simulink model "Architecture"  (R2020b)
settings: Solver=VariableStepAuto  StartTime=0.0  StopTime=10.0  RelTol=1e-3
undefined symbols (not defined in the file or in its folder): des, T
libraries: simulink x16
(part 1 of 6)
settings Model: Creator=James Webb  LastModifiedBy=James Webb

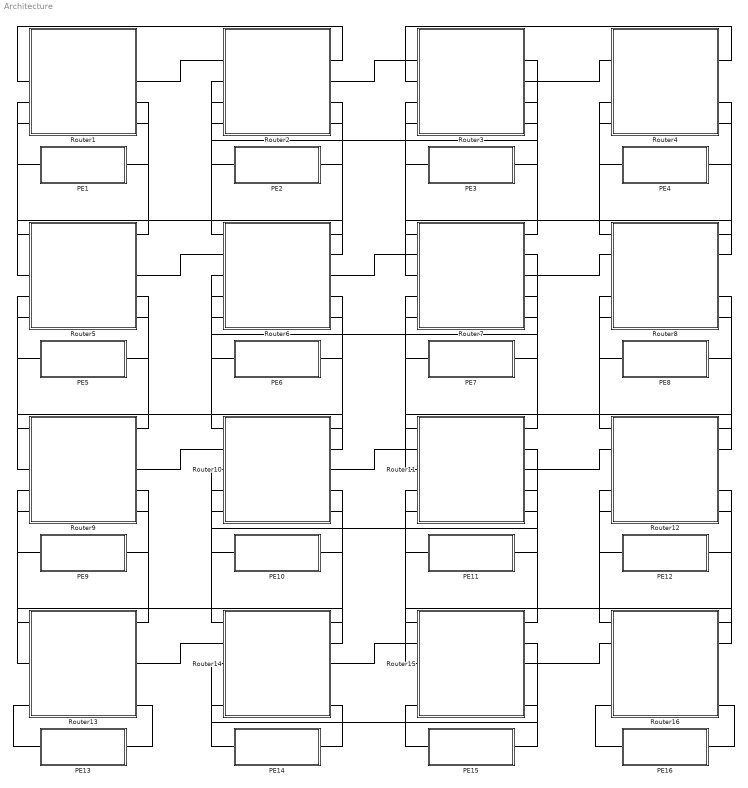
== system Architecture ==
  PE1 : Subsystem  mask{V=[4 16], P=ones(1,2)./2, SELECT=1, ME=1, D=5, SEED=100, tt=Periodic, MINU=10, MAXU=200, REGULAR=T, A=100, B=15, Inst='Inst1', Router='Mean1', Loss='Loss1', N='N1'}
      mask prompts: V "Traffic Pattern"; P "Probabilistic Pattern"; ME "Adress"; D "Startup time"; tt "Traffic Type"; MINU "Min"; MAXU "Max"; REGULAR "T"; A "Lambda 1"; B "Lambda 2"; Inst "Instant delay"; Router "Mean delay"; Loss "Instant number of lost flits"; N "Number of departed flits"
      mask init:
      | set_param([gcb '/Inst'],'VariableName',Inst)
      | set_param([gcb '/Router'],'VariableName',Router)
      | set_param([gcb '/Loss'],'VariableName',Loss)
      | set_param([gcb '/N'],'VariableName',N)
      | %V=[2 7 13];
      | %V=1:20;
      | %V=V(V~=ME);
      mask TypeOptions tt: Periodic | Uniform | MMPP
      mask Callback tt:
      | maskStr = get_param(gcb,'tt');
      | msk = Simulink.Mask.get(gcbh);
      | %p = msk.Parameters;
      | %
      | % P = msk.getParameter('MINU');
      | % U = msk.getParameter('MAXU');
      | % M = msk.getParameter('REGULAR');
      | 
      | P = msk.getDialogControl('Periodic');
      | U = msk.getDialogControl('Uniform');
      | M = msk.getDialogControl('MMPP');
      | 
      | % The pop-up menu is the first mask parameter.
      | %   Check the value selected in the pop-up
      | if strcmp(maskStr(1),'P'),
      | 
      |     % Set the visibility of both parameters on when
      |     %   User-defined is selected in the pop-up.
      |     %set_param(gcb,'MaskValues',{'Default','1','1'})
      |     %set_param(gcb,'MaskVisibilities','off'),
      |     SELECT = 1;
      |     P.Visible= 'on';
      |     U.Visible= 'off';
      |     M.Visible= 'off';
      | 
      | elseif strcmp(maskStr(1),'U'),
      |     P.Visible= 'off';
      |     U.Visible= 'on';
      |     M.Visible= 'off';
      | 
      |     SELECT = 2;
      | else
      |     P.Visible= 'off';
      |     U.Visible= 'off';
      |     M.Visible= 'on';
      | 
      |     SELECT = 3;
      | end
      mask DialogControl DescGroupVar Prompt: Processing Element
      mask DialogControl DescTextVar Prompt: Generates traffic from a given adress using one of three possible traffic patterns: Periodic, Uniform and Markov Modulated Poisson Process.
      mask DialogControl Container8 Prompt: Traffic Routing
      mask DialogControl Container3 Prompt: Parameters
      mask DialogControl Uniform Prompt: Uniform
      mask DialogControl Periodic Prompt: Periodic
      mask DialogControl MMPP Prompt: MMPP
      mask DialogControl Container7 Prompt: Output Variables
  PE10 : Subsystem  mask{V=[3 15], P=ones(1,2)./2, SELECT=1, ME=10, D=5, SEED=100, tt=Periodic, MINU=10, MAXU=200, REGULAR=T, A=100, B=15, Inst='Inst10', Router='Mean10', Loss='Loss10', N='N10'}
      mask prompts: V "Traffic Pattern"; P "Probabilistic Pattern"; ME "Adress"; D "Startup time"; tt "Traffic Type"; MINU "Min"; MAXU "Max"; REGULAR "T"; A "Lambda 1"; B "Lambda 2"; Inst "Instant delay"; Router "Mean delay"; Loss "Instant number of lost flits"; N "Number of departed flits"
      mask init: same as Architecture/PE1
      mask TypeOptions tt: Periodic | Uniform | MMPP
      mask Callback tt:
      | maskStr = get_param(gcb,'tt');
      | msk = Simulink.Mask.get(gcbh);
      | %p = msk.Parameters;
      | %
      | % P = msk.getParameter('MINU');
      | % U = msk.getParameter('MAXU');
      | % M = msk.getParameter('REGULAR');
      | 
      | P = msk.getDialogControl('Periodic');
      | U = msk.getDialogControl('Uniform');
      | M = msk.getDialogControl('MMPP');
      | 
      | % The pop-up menu is the first mask parameter.
      | %   Check the value selected in the pop-up
      | if strcmp(maskStr(1),'P'),
      | 
      |     % Set the visibility of both parameters on when
      |     %   User-defined is selected in the pop-up.
      |     %set_param(gcb,'MaskValues',{'Default','1','1'})
      |     %set_param(gcb,'MaskVisibilities','off'),
      |     SELECT = 1;
      |     P.Visible= 'on';
      |     U.Visible= 'off';
      |     M.Visible= 'off';
      | 
      | elseif strcmp(maskStr(1),'U'),
      |     P.Visible= 'off';
      |     U.Visible= 'on';
      |     M.Visible= 'off';
      | 
      |     SELECT = 2;
      | else
      |     P.Visible= 'off';
      |     U.Visible= 'off';
      |     M.Visible= 'on';
      | 
      |     SELECT = 3;
      | end
      mask DialogControl DescGroupVar Prompt: Processing Element
      mask DialogControl DescTextVar Prompt: Generates traffic from a given adress using one of three possible traffic patterns: Periodic, Uniform and Markov Modulated Poisson Process.
      mask DialogControl Container8 Prompt: Traffic Routing
      mask DialogControl Container3 Prompt: Parameters
      mask DialogControl Uniform Prompt: Uniform
      mask DialogControl Periodic Prompt: Periodic
      mask DialogControl MMPP Prompt: MMPP
      mask DialogControl Container7 Prompt: Output Variables
  PE11 : Subsystem  mask{SELECT=1, ME=11, D=5, SEED=100, tt=Periodic, MINU=10, MAXU=200, REGULAR=T, A=100, B=15, Inst='Inst11', Router='Mean11', Loss='Loss11', N='N11'}
      mask prompts: ME "Adress"; D "Startup time"; tt "Traffic Type"; MINU "Min"; MAXU "Max"; REGULAR "T"; A "Lambda 1"; B "Lambda 2"; Inst "Instant delay"; Router "Mean delay"; Loss "Instant number of lost flits"; N "Number of departed flits"
      mask init: same as Architecture/PE1
      mask TypeOptions tt: Periodic | Uniform | MMPP
      mask Callback tt:
      | maskStr = get_param(gcb,'tt');
      | msk = Simulink.Mask.get(gcbh);
      | %p = msk.Parameters;
      | %
      | % P = msk.getParameter('MINU');
      | % U = msk.getParameter('MAXU');
      | % M = msk.getParameter('REGULAR');
      | 
      | P = msk.getDialogControl('Periodic');
      | U = msk.getDialogControl('Uniform');
      | M = msk.getDialogControl('MMPP');
      | 
      | % The pop-up menu is the first mask parameter.
      | %   Check the value selected in the pop-up
      | if strcmp(maskStr(1),'P'),
      | 
      |     % Set the visibility of both parameters on when
      |     %   User-defined is selected in the pop-up.
      |     %set_param(gcb,'MaskValues',{'Default','1','1'})
      |     %set_param(gcb,'MaskVisibilities','off'),
      |     SELECT = 1;
      |     P.Visible= 'on';
      |     U.Visible= 'off';
      |     M.Visible= 'off';
      | 
      | elseif strcmp(maskStr(1),'U'),
      |     P.Visible= 'off';
      |     U.Visible= 'on';
      |     M.Visible= 'off';
      | 
      |     SELECT = 2;
      | else
      |     P.Visible= 'off';
      |     U.Visible= 'off';
      |     M.Visible= 'on';
      | 
      |     SELECT = 3;
      | end
      mask DialogControl DescGroupVar Prompt: Processing Element
      mask DialogControl DescTextVar Prompt: Generates traffic from a given adress using one of three possible traffic patterns: Periodic, Uniform and Markov Modulated Poisson Process.
      mask DialogControl Container8 Prompt: Traffic Routing
      mask DialogControl Container3 Prompt: Parameters
      mask DialogControl Uniform Prompt: Uniform
      mask DialogControl Periodic Prompt: Periodic
      mask DialogControl MMPP Prompt: MMPP
      mask DialogControl Container7 Prompt: Output Variables
  PE12 : Subsystem  mask{SELECT=1, ME=12, D=5, SEED=100, tt=Periodic, MINU=10, MAXU=200, REGULAR=T, A=100, B=15, Inst='Inst12', Router='Mean12', Loss='Loss12', N='N12'}
      mask prompts: ME "Adress"; D "Startup time"; tt "Traffic Type"; MINU "Min"; MAXU "Max"; REGULAR "T"; A "Lambda 1"; B "Lambda 2"; Inst "Instant delay"; Router "Mean delay"; Loss "Instant number of lost flits"; N "Number of departed flits"
      mask init: same as Architecture/PE1
      mask TypeOptions tt: Periodic | Uniform | MMPP
      mask Callback tt:
      | maskStr = get_param(gcb,'tt');
      | msk = Simulink.Mask.get(gcbh);
      | %p = msk.Parameters;
      | %
      | % P = msk.getParameter('MINU');
      | % U = msk.getParameter('MAXU');
      | % M = msk.getParameter('REGULAR');
      | 
      | P = msk.getDialogControl('Periodic');
      | U = msk.getDialogControl('Uniform');
      | M = msk.getDialogControl('MMPP');
      | 
      | % The pop-up menu is the first mask parameter.
      | %   Check the value selected in the pop-up
      | if strcmp(maskStr(1),'P'),
      | 
      |     % Set the visibility of both parameters on when
      |     %   User-defined is selected in the pop-up.
      |     %set_param(gcb,'MaskValues',{'Default','1','1'})
      |     %set_param(gcb,'MaskVisibilities','off'),
      |     SELECT = 1;
      |     P.Visible= 'on';
      |     U.Visible= 'off';
      |     M.Visible= 'off';
      | 
      | elseif strcmp(maskStr(1),'U'),
      |     P.Visible= 'off';
      |     U.Visible= 'on';
      |     M.Visible= 'off';
      | 
      |     SELECT = 2;
      | else
      |     P.Visible= 'off';
      |     U.Visible= 'off';
      |     M.Visible= 'on';
      | 
      |     SELECT = 3;
      | end
      mask DialogControl DescGroupVar Prompt: Processing Element
      mask DialogControl DescTextVar Prompt: Generates traffic from a given adress using one of three possible traffic patterns: Periodic, Uniform and Markov Modulated Poisson Process.
      mask DialogControl Container8 Prompt: Traffic Routing
      mask DialogControl Container3 Prompt: Parameters
      mask DialogControl Uniform Prompt: Uniform
      mask DialogControl Periodic Prompt: Periodic
      mask DialogControl MMPP Prompt: MMPP
      mask DialogControl Container7 Prompt: Output Variables
  PE13 : Subsystem  mask{SELECT=1, ME=13, D=5, SEED=100, tt=Periodic, MINU=10, MAXU=200, REGULAR=T, A=100, B=15, Inst='Inst13', Router='Mean13', Loss='Loss13', N='N13'}
      mask prompts: ME "Adress"; D "Startup time"; tt "Traffic Type"; MINU "Min"; MAXU "Max"; REGULAR "T"; A "Lambda 1"; B "Lambda 2"; Inst "Instant delay"; Router "Mean delay"; Loss "Instant number of lost flits"; N "Number of departed flits"
      mask init: same as Architecture/PE1
      mask TypeOptions tt: Periodic | Uniform | MMPP
      mask Callback tt:
      | maskStr = get_param(gcb,'tt');
      | msk = Simulink.Mask.get(gcbh);
      | %p = msk.Parameters;
      | %
      | % P = msk.getParameter('MINU');
      | % U = msk.getParameter('MAXU');
      | % M = msk.getParameter('REGULAR');
      | 
      | P = msk.getDialogControl('Periodic');
      | U = msk.getDialogControl('Uniform');
      | M = msk.getDialogControl('MMPP');
      | 
      | % The pop-up menu is the first mask parameter.
      | %   Check the value selected in the pop-up
      | if strcmp(maskStr(1),'P'),
      | 
      |     % Set the visibility of both parameters on when
      |     %   User-defined is selected in the pop-up.
      |     %set_param(gcb,'MaskValues',{'Default','1','1'})
      |     %set_param(gcb,'MaskVisibilities','off'),
      |     SELECT = 1;
      |     P.Visible= 'on';
      |     U.Visible= 'off';
      |     M.Visible= 'off';
      | 
      | elseif strcmp(maskStr(1),'U'),
      |     P.Visible= 'off';
      |     U.Visible= 'on';
      |     M.Visible= 'off';
      | 
      |     SELECT = 2;
      | else
      |     P.Visible= 'off';
      |     U.Visible= 'off';
      |     M.Visible= 'on';
      | 
      |     SELECT = 3;
      | end
      mask DialogControl DescGroupVar Prompt: Processing Element
      mask DialogControl DescTextVar Prompt: Generates traffic from a given adress using one of three possible traffic patterns: Periodic, Uniform and Markov Modulated Poisson Process.
      mask DialogControl Container8 Prompt: Traffic Routing
      mask DialogControl Container3 Prompt: Parameters
      mask DialogControl Uniform Prompt: Uniform
      mask DialogControl Periodic Prompt: Periodic
      mask DialogControl MMPP Prompt: MMPP
      mask DialogControl Container7 Prompt: Output Variables
  PE14 : Subsystem  mask{V=[4 8], P=ones(1,2)./2, SELECT=1, ME=14, D=5, SEED=100, tt=Periodic, MINU=10, MAXU=200, REGULAR=T, A=100, B=15, Inst='Inst14', Router='Mean14', Loss='Loss14', N='N14'}
      mask prompts: V "Traffic Pattern"; P "Probabilistic Pattern"; ME "Adress"; D "Startup time"; tt "Traffic Type"; MINU "Min"; MAXU "Max"; REGULAR "T"; A "Lambda 1"; B "Lambda 2"; Inst "Instant delay"; Router "Mean delay"; Loss "Instant number of lost flits"; N "Number of departed flits"
      mask init: same as Architecture/PE1
      mask TypeOptions tt: Periodic | Uniform | MMPP
      mask Callback tt:
      | maskStr = get_param(gcb,'tt');
      | msk = Simulink.Mask.get(gcbh);
      | %p = msk.Parameters;
      | %
      | % P = msk.getParameter('MINU');
      | % U = msk.getParameter('MAXU');
      | % M = msk.getParameter('REGULAR');
      | 
      | P = msk.getDialogControl('Periodic');
      | U = msk.getDialogControl('Uniform');
      | M = msk.getDialogControl('MMPP');
      | 
      | % The pop-up menu is the first mask parameter.
      | %   Check the value selected in the pop-up
      | if strcmp(maskStr(1),'P'),
      | 
      |     % Set the visibility of both parameters on when
      |     %   User-defined is selected in the pop-up.
      |     %set_param(gcb,'MaskValues',{'Default','1','1'})
      |     %set_param(gcb,'MaskVisibilities','off'),
      |     SELECT = 1;
      |     P.Visible= 'on';
      |     U.Visible= 'off';
      |     M.Visible= 'off';
      | 
      | elseif strcmp(maskStr(1),'U'),
      |     P.Visible= 'off';
      |     U.Visible= 'on';
      |     M.Visible= 'off';
      | 
      |     SELECT = 2;
      | else
      |     P.Visible= 'off';
      |     U.Visible= 'off';
      |     M.Visible= 'on';
      | 
      |     SELECT = 3;
      | end
      mask DialogControl DescGroupVar Prompt: Processing Element
      mask DialogControl DescTextVar Prompt: Generates traffic from a given adress using one of three possible traffic patterns: Periodic, Uniform and Markov Modulated Poisson Process.
      mask DialogControl Container8 Prompt: Traffic Routing
      mask DialogControl Container3 Prompt: Parameters
      mask DialogControl Uniform Prompt: Uniform
      mask DialogControl Periodic Prompt: Periodic
      mask DialogControl MMPP Prompt: MMPP
      mask DialogControl Container7 Prompt: Output Variables
  PE15 : Subsystem  mask{SELECT=1, DST1=[2], ME=15, D=5, SEED=100, tt=Periodic, MINU=10, MAXU=200, REGULAR=T, A=100, B=15, Inst='Inst15', Router='Mean15', Loss='Loss15', N='N15'}
      mask prompts: DST1 "Destino"; ME "Adress"; D "Startup time"; tt "Traffic Type"; MINU "Min"; MAXU "Max"; REGULAR "T"; A "Lambda 1"; B "Lambda 2"; Inst "Instant delay"; Router "Mean delay"; Loss "Instant number of lost flits"; N "Number of departed flits"
      mask init: same as Architecture/PE1
      mask TypeOptions tt: Periodic | Uniform | MMPP
      mask Callback tt:
      | maskStr = get_param(gcb,'tt');
      | msk = Simulink.Mask.get(gcbh);
      | %p = msk.Parameters;
      | %
      | % P = msk.getParameter('MINU');
      | % U = msk.getParameter('MAXU');
      | % M = msk.getParameter('REGULAR');
      | 
      | P = msk.getDialogControl('Periodic');
      | U = msk.getDialogControl('Uniform');
      | M = msk.getDialogControl('MMPP');
      | 
      | % The pop-up menu is the first mask parameter.
      | %   Check the value selected in the pop-up
      | if strcmp(maskStr(1),'P'),
      | 
      |     % Set the visibility of both parameters on when
      |     %   User-defined is selected in the pop-up.
      |     %set_param(gcb,'MaskValues',{'Default','1','1'})
      |     %set_param(gcb,'MaskVisibilities','off'),
      |     SELECT = 1;
      |     P.Visible= 'on';
      |     U.Visible= 'off';
      |     M.Visible= 'off';
      | 
      | elseif strcmp(maskStr(1),'U'),
      |     P.Visible= 'off';
      |     U.Visible= 'on';
      |     M.Visible= 'off';
      | 
      |     SELECT = 2;
      | else
      |     P.Visible= 'off';
      |     U.Visible= 'off';
      |     M.Visible= 'on';
      | 
      |     SELECT = 3;
      | end
      mask DialogControl DescGroupVar Prompt: Processing Element
      mask DialogControl DescTextVar Prompt: Generates traffic from a given adress using one of three possible traffic patterns: Periodic, Uniform and Markov Modulated Poisson Process.
      mask DialogControl Container8 Prompt: Traffic Routing
      mask DialogControl Container3 Prompt: Parameters
      mask DialogControl Uniform Prompt: Uniform
      mask DialogControl Periodic Prompt: Periodic
      mask DialogControl MMPP Prompt: MMPP
      mask DialogControl Container7 Prompt: Output Variables
  PE16 : Subsystem  mask{SELECT=1, DST1=[2], ME=16, D=5, SEED=100, tt=Periodic, MINU=10, MAXU=200, REGULAR=T, A=100, B=15, Inst='Inst16', Router='Mean16', Loss='Loss16', N='N16'}
      mask prompts: DST1 "Destino"; ME "Adress"; D "Startup time"; tt "Traffic Type"; MINU "Min"; MAXU "Max"; REGULAR "T"; A "Lambda 1"; B "Lambda 2"; Inst "Instant delay"; Router "Mean delay"; Loss "Instant number of lost flits"; N "Number of departed flits"
      mask init: same as Architecture/PE1
      mask TypeOptions tt: Periodic | Uniform | MMPP
      mask Callback tt:
      | maskStr = get_param(gcb,'tt');
      | msk = Simulink.Mask.get(gcbh);
      | %p = msk.Parameters;
      | %
      | % P = msk.getParameter('MINU');
      | % U = msk.getParameter('MAXU');
      | % M = msk.getParameter('REGULAR');
      | 
      | P = msk.getDialogControl('Periodic');
      | U = msk.getDialogControl('Uniform');
      | M = msk.getDialogControl('MMPP');
      | 
      | % The pop-up menu is the first mask parameter.
      | %   Check the value selected in the pop-up
      | if strcmp(maskStr(1),'P'),
      | 
      |     % Set the visibility of both parameters on when
      |     %   User-defined is selected in the pop-up.
      |     %set_param(gcb,'MaskValues',{'Default','1','1'})
      |     %set_param(gcb,'MaskVisibilities','off'),
      |     SELECT = 1;
      |     P.Visible= 'on';
      |     U.Visible= 'off';
      |     M.Visible= 'off';
      | 
      | elseif strcmp(maskStr(1),'U'),
      |     P.Visible= 'off';
      |     U.Visible= 'on';
      |     M.Visible= 'off';
      | 
      |     SELECT = 2;
      | else
      |     P.Visible= 'off';
      |     U.Visible= 'off';
      |     M.Visible= 'on';
      | 
      |     SELECT = 3;
      | end
      mask DialogControl DescGroupVar Prompt: Processing Element
      mask DialogControl DescTextVar Prompt: Generates traffic from a given adress using one of three possible traffic patterns: Periodic, Uniform and Markov Modulated Poisson Process.
      mask DialogControl Container8 Prompt: Traffic Routing
      mask DialogControl Container3 Prompt: Parameters
      mask DialogControl Uniform Prompt: Uniform
      mask DialogControl Periodic Prompt: Periodic
      mask DialogControl MMPP Prompt: MMPP
      mask DialogControl Container7 Prompt: Output Variables
  PE2 : Subsystem  mask{V=[3 7 8 9 15], P=ones(1,5)./5, SELECT=1, ME=2, D=5, SEED=100, tt=Periodic, MINU=10, MAXU=200, REGULAR=T, A=100, B=15, Inst='Inst2', Router='Mean2', Loss='Loss2', N='N2'}
      mask prompts: V "Traffic Pattern"; P "Probabilistic Pattern"; ME "Adress"; D "Startup time"; tt "Traffic Type"; MINU "Min"; MAXU "Max"; REGULAR "T"; A "Lambda 1"; B "Lambda 2"; Inst "Instant delay"; Router "Mean delay"; Loss "Instant number of lost flits"; N "Number of departed flits"
      mask init: same as Architecture/PE1
      mask TypeOptions tt: Periodic | Uniform | MMPP
      mask Callback tt:
      | maskStr = get_param(gcb,'tt');
      | msk = Simulink.Mask.get(gcbh);
      | %p = msk.Parameters;
      | %
      | % P = msk.getParameter('MINU');
      | % U = msk.getParameter('MAXU');
      | % M = msk.getParameter('REGULAR');
      | 
      | P = msk.getDialogControl('Periodic');
      | U = msk.getDialogControl('Uniform');
      | M = msk.getDialogControl('MMPP');
      | 
      | % The pop-up menu is the first mask parameter.
      | %   Check the value selected in the pop-up
      | if strcmp(maskStr(1),'P'),
      | 
      |     % Set the visibility of both parameters on when
      |     %   User-defined is selected in the pop-up.
      |     %set_param(gcb,'MaskValues',{'Default','1','1'})
      |     %set_param(gcb,'MaskVisibilities','off'),
      |     SELECT = 1;
      |     P.Visible= 'on';
      |     U.Visible= 'off';
      |     M.Visible= 'off';
      | 
      | elseif strcmp(maskStr(1),'U'),
      |     P.Visible= 'off';
      |     U.Visible= 'on';
      |     M.Visible= 'off';
      | 
      |     SELECT = 2;
      | else
      |     P.Visible= 'off';
      |     U.Visible= 'off';
      |     M.Visible= 'on';
      | 
      |     SELECT = 3;
      | end
      mask DialogControl DescGroupVar Prompt: Processing Element
      mask DialogControl DescTextVar Prompt: Generates traffic from a given adress using one of three possible traffic patterns: Periodic, Uniform and Markov Modulated Poisson Process.
      mask DialogControl Container8 Prompt: Traffic Routing
      mask DialogControl Container3 Prompt: Parameters
      mask DialogControl Uniform Prompt: Uniform
      mask DialogControl Periodic Prompt: Periodic
      mask DialogControl MMPP Prompt: MMPP
      mask DialogControl Container7 Prompt: Output Variables
  PE3 : Subsystem  mask{SELECT=1, DST1=[2], ME=3, D=5, SEED=100, tt=Periodic, MINU=10, MAXU=200, REGULAR=T, A=100, B=15, Inst='Inst3', Router='Mean3', Loss='Loss3', N='N3'}
      mask prompts: DST1 "Destino"; ME "Adress"; D "Startup time"; tt "Traffic Type"; MINU "Min"; MAXU "Max"; REGULAR "T"; A "Lambda 1"; B "Lambda 2"; Inst "Instant delay"; Router "Mean delay"; Loss "Instant number of lost flits"; N "Number of departed flits"
      mask init: same as Architecture/PE1
      mask TypeOptions tt: Periodic | Uniform | MMPP
      mask Callback tt:
      | maskStr = get_param(gcb,'tt');
      | msk = Simulink.Mask.get(gcbh);
      | %p = msk.Parameters;
      | %
      | % P = msk.getParameter('MINU');
      | % U = msk.getParameter('MAXU');
      | % M = msk.getParameter('REGULAR');
      | 
      | P = msk.getDialogControl('Periodic');
      | U = msk.getDialogControl('Uniform');
      | M = msk.getDialogControl('MMPP');
      | 
      | % The pop-up menu is the first mask parameter.
      | %   Check the value selected in the pop-up
      | if strcmp(maskStr(1),'P'),
      | 
      |     % Set the visibility of both parameters on when
      |     %   User-defined is selected in the pop-up.
      |     %set_param(gcb,'MaskValues',{'Default','1','1'})
      |     %set_param(gcb,'MaskVisibilities','off'),
      |     SELECT = 1;
      |     P.Visible= 'on';
      |     U.Visible= 'off';
      |     M.Visible= 'off';
      | 
      | elseif strcmp(maskStr(1),'U'),
      |     P.Visible= 'off';
      |     U.Visible= 'on';
      |     M.Visible= 'off';
      | 
      |     SELECT = 2;
      | else
      |     P.Visible= 'off';
      |     U.Visible= 'off';
      |     M.Visible= 'on';
      | 
      |     SELECT = 3;
      | end
      mask DialogControl DescGroupVar Prompt: Processing Element
      mask DialogControl DescTextVar Prompt: Generates traffic from a given adress using one of three possible traffic patterns: Periodic, Uniform and Markov Modulated Poisson Process.
      mask DialogControl Container8 Prompt: Traffic Routing
      mask DialogControl Container3 Prompt: Parameters
      mask DialogControl Uniform Prompt: Uniform
      mask DialogControl Periodic Prompt: Periodic
      mask DialogControl MMPP Prompt: MMPP
      mask DialogControl Container7 Prompt: Output Variables
  PE4 : Subsystem  mask{SELECT=1, DST1=[7], ME=4, D=5, SEED=100, tt=Periodic, MINU=10, MAXU=200, REGULAR=T, A=100, B=15, Inst='Inst4', Router='Mean4', Loss='Loss4', N='N4'}
      mask prompts: DST1 "Destino"; ME "Adress"; D "Startup time"; tt "Traffic Type"; MINU "Min"; MAXU "Max"; REGULAR "T"; A "Lambda 1"; B "Lambda 2"; Inst "Instant delay"; Router "Mean delay"; Loss "Instant number of lost flits"; N "Number of departed flits"
      mask init: same as Architecture/PE1
      mask TypeOptions tt: Periodic | Uniform | MMPP
      mask Callback tt:
      | maskStr = get_param(gcb,'tt');
      | msk = Simulink.Mask.get(gcbh);
      | %p = msk.Parameters;
      | %
      | % P = msk.getParameter('MINU');
      | % U = msk.getParameter('MAXU');
      | % M = msk.getParameter('REGULAR');
      | 
      | P = msk.getDialogControl('Periodic');
      | U = msk.getDialogControl('Uniform');
      | M = msk.getDialogControl('MMPP');
      | 
      | % The pop-up menu is the first mask parameter.
      | %   Check the value selected in the pop-up
      | if strcmp(maskStr(1),'P'),
      | 
      |     % Set the visibility of both parameters on when
      |     %   User-defined is selected in the pop-up.
      |     %set_param(gcb,'MaskValues',{'Default','1','1'})
      |     %set_param(gcb,'MaskVisibilities','off'),
      |     SELECT = 1;
      |     P.Visible= 'on';
      |     U.Visible= 'off';
      |     M.Visible= 'off';
      | 
      | elseif strcmp(maskStr(1),'U'),
      |     P.Visible= 'off';
      |     U.Visible= 'on';
      |     M.Visible= 'off';
      | 
      |     SELECT = 2;
      | else
      |     P.Visible= 'off';
      |     U.Visible= 'off';
      |     M.Visible= 'on';
      | 
      |     SELECT = 3;
      | end
      mask DialogControl DescGroupVar Prompt: Processing Element
      mask DialogControl DescTextVar Prompt: Generates traffic from a given adress using one of three possible traffic patterns: Periodic, Uniform and Markov Modulated Poisson Process.
      mask DialogControl Container8 Prompt: Traffic Routing
      mask DialogControl Container3 Prompt: Parameters
      mask DialogControl Uniform Prompt: Uniform
      mask DialogControl Periodic Prompt: Periodic
      mask DialogControl MMPP Prompt: MMPP
      mask DialogControl Container7 Prompt: Output Variables
  PE5 : Subsystem  mask{SELECT=1, ME=5, D=5, SEED=100, tt=Periodic, MINU=10, MAXU=200, REGULAR=T, A=100, B=15, Inst='Inst5', Router='Mean5', Loss='Loss5', N='N5'}
      mask prompts: ME "Adress"; D "Startup time"; tt "Traffic Type"; MINU "Min"; MAXU "Max"; REGULAR "T"; A "Lambda 1"; B "Lambda 2"; Inst "Instant delay"; Router "Mean delay"; Loss "Instant number of lost flits"; N "Number of departed flits"
      mask init: same as Architecture/PE1
      mask TypeOptions tt: Periodic | Uniform | MMPP
      mask Callback tt:
      | maskStr = get_param(gcb,'tt');
      | msk = Simulink.Mask.get(gcbh);
      | %p = msk.Parameters;
      | %
      | % P = msk.getParameter('MINU');
      | % U = msk.getParameter('MAXU');
      | % M = msk.getParameter('REGULAR');
      | 
      | P = msk.getDialogControl('Periodic');
      | U = msk.getDialogControl('Uniform');
      | M = msk.getDialogControl('MMPP');
      | 
      | % The pop-up menu is the first mask parameter.
      | %   Check the value selected in the pop-up
      | if strcmp(maskStr(1),'P'),
      | 
      |     % Set the visibility of both parameters on when
      |     %   User-defined is selected in the pop-up.
      |     %set_param(gcb,'MaskValues',{'Default','1','1'})
      |     %set_param(gcb,'MaskVisibilities','off'),
      |     SELECT = 1;
      |     P.Visible= 'on';
      |     U.Visible= 'off';
      |     M.Visible= 'off';
      | 
      | elseif strcmp(maskStr(1),'U'),
      |     P.Visible= 'off';
      |     U.Visible= 'on';
      |     M.Visible= 'off';
      | 
      |     SELECT = 2;
      | else
      |     P.Visible= 'off';
      |     U.Visible= 'off';
      |     M.Visible= 'on';
      | 
      |     SELECT = 3;
      | end
      mask DialogControl DescGroupVar Prompt: Processing Element
      mask DialogControl DescTextVar Prompt: Generates traffic from a given adress using one of three possible traffic patterns: Periodic, Uniform and Markov Modulated Poisson Process.
      mask DialogControl Container8 Prompt: Traffic Routing
      mask DialogControl Container3 Prompt: Parameters
      mask DialogControl Uniform Prompt: Uniform
      mask DialogControl Periodic Prompt: Periodic
      mask DialogControl MMPP Prompt: MMPP
      mask DialogControl Container7 Prompt: Output Variables
  PE6 : Subsystem  mask{SELECT=1, DST1=[3], ME=6, D=5, SEED=100, tt=Periodic, MINU=10, MAXU=200, REGULAR=T, A=100, B=15, Inst='Inst6', Router='Mean6', Loss='Loss6', N='N6'}
      mask prompts: DST1 "Destino"; ME "Adress"; D "Startup time"; tt "Traffic Type"; MINU "Min"; MAXU "Max"; REGULAR "T"; A "Lambda 1"; B "Lambda 2"; Inst "Instant delay"; Router "Mean delay"; Loss "Instant number of lost flits"; N "Number of departed flits"
      mask init: same as Architecture/PE1
      mask TypeOptions tt: Periodic | Uniform | MMPP
      mask Callback tt:
      | maskStr = get_param(gcb,'tt');
      | msk = Simulink.Mask.get(gcbh);
      | %p = msk.Parameters;
      | %
      | % P = msk.getParameter('MINU');
      | % U = msk.getParameter('MAXU');
      | % M = msk.getParameter('REGULAR');
      | 
      | P = msk.getDialogControl('Periodic');
      | U = msk.getDialogControl('Uniform');
      | M = msk.getDialogControl('MMPP');
      | 
      | % The pop-up menu is the first mask parameter.
      | %   Check the value selected in the pop-up
      | if strcmp(maskStr(1),'P'),
      | 
      |     % Set the visibility of both parameters on when
      |     %   User-defined is selected in the pop-up.
      |     %set_param(gcb,'MaskValues',{'Default','1','1'})
      |     %set_param(gcb,'MaskVisibilities','off'),
      |     SELECT = 1;
      |     P.Visible= 'on';
      |     U.Visible= 'off';
      |     M.Visible= 'off';
      | 
      | elseif strcmp(maskStr(1),'U'),
      |     P.Visible= 'off';
      |     U.Visible= 'on';
      |     M.Visible= 'off';
      | 
      |     SELECT = 2;
      | else
      |     P.Visible= 'off';
      |     U.Visible= 'off';
      |     M.Visible= 'on';
      | 
      |     SELECT = 3;
      | end
      mask DialogControl DescGroupVar Prompt: Processing Element
      mask DialogControl DescTextVar Prompt: Generates traffic from a given adress using one of three possible traffic patterns: Periodic, Uniform and Markov Modulated Poisson Process.
      mask DialogControl Container8 Prompt: Traffic Routing
      mask DialogControl Container3 Prompt: Parameters
      mask DialogControl Uniform Prompt: Uniform
      mask DialogControl Periodic Prompt: Periodic
      mask DialogControl MMPP Prompt: MMPP
      mask DialogControl Container7 Prompt: Output Variables
  PE7 : Subsystem  mask{V=[4 9], P=ones(1,2)./2, SELECT=1, ME=7, D=5, SEED=100, tt=Periodic, MINU=10, MAXU=200, REGULAR=T, A=100, B=15, Inst='Inst7', Router='Mean7', Loss='Loss7', N='N7'}
      mask prompts: V "Traffic Pattern"; P "Probabilistic Pattern"; ME "Adress"; D "Startup time"; tt "Traffic Type"; MINU "Min"; MAXU "Max"; REGULAR "T"; A "Lambda 1"; B "Lambda 2"; Inst "Instant delay"; Router "Mean delay"; Loss "Instant number of lost flits"; N "Number of departed flits"
      mask init: same as Architecture/PE1
      mask TypeOptions tt: Periodic | Uniform | MMPP
      mask Callback tt:
      | maskStr = get_param(gcb,'tt');
      | msk = Simulink.Mask.get(gcbh);
      | %p = msk.Parameters;
      | %
      | % P = msk.getParameter('MINU');
      | % U = msk.getParameter('MAXU');
      | % M = msk.getParameter('REGULAR');
      | 
      | P = msk.getDialogControl('Periodic');
      | U = msk.getDialogControl('Uniform');
      | M = msk.getDialogControl('MMPP');
      | 
      | % The pop-up menu is the first mask parameter.
      | %   Check the value selected in the pop-up
      | if strcmp(maskStr(1),'P'),
      | 
      |     % Set the visibility of both parameters on when
      |     %   User-defined is selected in the pop-up.
      |     %set_param(gcb,'MaskValues',{'Default','1','1'})
      |     %set_param(gcb,'MaskVisibilities','off'),
      |     SELECT = 1;
      |     P.Visible= 'on';
      |     U.Visible= 'off';
      |     M.Visible= 'off';
      | 
      | elseif strcmp(maskStr(1),'U'),
      |     P.Visible= 'off';
      |     U.Visible= 'on';
      |     M.Visible= 'off';
      | 
      |     SELECT = 2;
      | else
      |     P.Visible= 'off';
      |     U.Visible= 'off';
      |     M.Visible= 'on';
      | 
      |     SELECT = 3;
      | end
      mask DialogControl DescGroupVar Prompt: Processing Element
      mask DialogControl DescTextVar Prompt: Generates traffic from a given adress using one of three possible traffic patterns: Periodic, Uniform and Markov Modulated Poisson Process.
      mask DialogControl Container8 Prompt: Traffic Routing
      mask DialogControl Container3 Prompt: Parameters
      mask DialogControl Uniform Prompt: Uniform
      mask DialogControl Periodic Prompt: Periodic
      mask DialogControl MMPP Prompt: MMPP
      mask DialogControl Container7 Prompt: Output Variables
  PE8 : Subsystem  mask{V=[10 15 16], P=ones(1,3)./3, SELECT=1, ME=8, D=5, SEED=100, tt=Periodic, MINU=10, MAXU=200, REGULAR=T, A=100, B=15, Inst='Inst8', Router='Mean8', Loss='Loss8', N='N8'}
      mask prompts: V "Traffic Pattern"; P "Probabilistic Pattern"; ME "Adress"; D "Startup time"; tt "Traffic Type"; MINU "Min"; MAXU "Max"; REGULAR "T"; A "Lambda 1"; B "Lambda 2"; Inst "Instant delay"; Router "Mean delay"; Loss "Instant number of lost flits"; N "Number of departed flits"
      mask init: same as Architecture/PE1
      mask TypeOptions tt: Periodic | Uniform | MMPP
      mask Callback tt:
      | maskStr = get_param(gcb,'tt');
      | msk = Simulink.Mask.get(gcbh);
      | %p = msk.Parameters;
      | %
      | % P = msk.getParameter('MINU');
      | % U = msk.getParameter('MAXU');
      | % M = msk.getParameter('REGULAR');
      | 
      | P = msk.getDialogControl('Periodic');
      | U = msk.getDialogControl('Uniform');
      | M = msk.getDialogControl('MMPP');
      | 
      | % The pop-up menu is the first mask parameter.
      | %   Check the value selected in the pop-up
      | if strcmp(maskStr(1),'P'),
      | 
      |     % Set the visibility of both parameters on when
      |     %   User-defined is selected in the pop-up.
      |     %set_param(gcb,'MaskValues',{'Default','1','1'})
      |     %set_param(gcb,'MaskVisibilities','off'),
      |     SELECT = 1;
      |     P.Visible= 'on';
      |     U.Visible= 'off';
      |     M.Visible= 'off';
      | 
      | elseif strcmp(maskStr(1),'U'),
      |     P.Visible= 'off';
      |     U.Visible= 'on';
      |     M.Visible= 'off';
      | 
      |     SELECT = 2;
      | else
      |     P.Visible= 'off';
      |     U.Visible= 'off';
      |     M.Visible= 'on';
      | 
      |     SELECT = 3;
      | end
      mask DialogControl DescGroupVar Prompt: Processing Element
      mask DialogControl DescTextVar Prompt: Generates traffic from a given adress using one of three possible traffic patterns: Periodic, Uniform and Markov Modulated Poisson Process.
      mask DialogControl Container8 Prompt: Traffic Routing
      mask DialogControl Container3 Prompt: Parameters
      mask DialogControl Uniform Prompt: Uniform
      mask DialogControl Periodic Prompt: Periodic
      mask DialogControl MMPP Prompt: MMPP
      mask DialogControl Container7 Prompt: Output Variables
  PE9 : Subsystem  mask{V=[2 15], P=ones(1,2)./2, SELECT=1, ME=9, D=5, SEED=100, tt=Periodic, MINU=10, MAXU=200, REGULAR=T, A=100, B=15, Inst='Inst9', Router='Mean9', Loss='Loss9', N='N9'}
      mask prompts: V "Traffic Pattern"; P "Probabilistic Pattern"; ME "Adress"; D "Startup time"; tt "Traffic Type"; MINU "Min"; MAXU "Max"; REGULAR "T"; A "Lambda 1"; B "Lambda 2"; Inst "Instant delay"; Router "Mean delay"; Loss "Instant number of lost flits"; N "Number of departed flits"
      mask init: same as Architecture/PE1
      mask TypeOptions tt: Periodic | Uniform | MMPP
      mask Callback tt:
      | maskStr = get_param(gcb,'tt');
      | msk = Simulink.Mask.get(gcbh);
      | %p = msk.Parameters;
      | %
      | % P = msk.getParameter('MINU');
      | % U = msk.getParameter('MAXU');
      | % M = msk.getParameter('REGULAR');
      | 
      | P = msk.getDialogControl('Periodic');
      | U = msk.getDialogControl('Uniform');
      | M = msk.getDialogControl('MMPP');
      | 
      | % The pop-up menu is the first mask parameter.
      | %   Check the value selected in the pop-up
      | if strcmp(maskStr(1),'P'),
      | 
      |     % Set the visibility of both parameters on when
      |     %   User-defined is selected in the pop-up.
      |     %set_param(gcb,'MaskValues',{'Default','1','1'})
      |     %set_param(gcb,'MaskVisibilities','off'),
      |     SELECT = 1;
      |     P.Visible= 'on';
      |     U.Visible= 'off';
      |     M.Visible= 'off';
      | 
      | elseif strcmp(maskStr(1),'U'),
      |     P.Visible= 'off';
      |     U.Visible= 'on';
      |     M.Visible= 'off';
      | 
      |     SELECT = 2;
      | else
      |     P.Visible= 'off';
      |     U.Visible= 'off';
      |     M.Visible= 'on';
      | 
      |     SELECT = 3;
      | end
      mask DialogControl DescGroupVar Prompt: Processing Element
      mask DialogControl DescTextVar Prompt: Generates traffic from a given adress using one of three possible traffic patterns: Periodic, Uniform and Markov Modulated Poisson Process.
      mask DialogControl Container8 Prompt: Traffic Routing
      mask DialogControl Container3 Prompt: Parameters
      mask DialogControl Uniform Prompt: Uniform
      mask DialogControl Periodic Prompt: Periodic
      mask DialogControl MMPP Prompt: MMPP
      mask DialogControl Container7 Prompt: Output Variables
  Router1 : Subsystem  mask{ME=1, C=1, D=1, F=1, S=1e-6}
      mask prompts: ME "Router index"; C "Input FIFO size in flits"; D "Routing and arbitration delay"; F "Clock Frequency"; S "Standard Deviation"
      mask DialogControl DescGroupVar Prompt: XY Router
      mask DialogControl DescTextVar Prompt: 5 Port router with the XY routing algorithm.
  Router10 : Subsystem  mask{ME=10, C=1, D=1, F=1, S=1e-6}
      mask prompts: ME "Router index"; C "Input FIFO size in flits"; D "Routing and arbitration delay"; F "Clock Frequency"; S "Standard Deviation"
      mask DialogControl DescGroupVar Prompt: XY Router
      mask DialogControl DescTextVar Prompt: 5 Port router with the XY routing algorithm.
  Router11 : Subsystem  mask{ME=11, C=1, D=1, F=1, S=1e-6}
      mask prompts: ME "Router index"; C "Input FIFO size in flits"; D "Routing and arbitration delay"; F "Clock Frequency"; S "Standard Deviation"
      mask DialogControl DescGroupVar Prompt: XY Router
      mask DialogControl DescTextVar Prompt: 5 Port router with the XY routing algorithm.
  Router12 : Subsystem  mask{ME=12, C=1, D=1, F=1, S=1e-6}
      mask prompts: ME "Router index"; C "Input FIFO size in flits"; D "Routing and arbitration delay"; F "Clock Frequency"; S "Standard Deviation"
      mask DialogControl DescGroupVar Prompt: XY Router
      mask DialogControl DescTextVar Prompt: 5 Port router with the XY routing algorithm.
  Router13 : Subsystem  mask{ME=13, C=1, D=1, F=1, S=1e-6}
      mask prompts: ME "Router index"; C "Input FIFO size in flits"; D "Routing and arbitration delay"; F "Clock Frequency"; S "Standard Deviation"
      mask DialogControl DescGroupVar Prompt: XY Router
      mask DialogControl DescTextVar Prompt: 5 Port router with the XY routing algorithm.
  Router14 : Subsystem  mask{ME=14, C=1, D=1, F=1, S=1e-6}
      mask prompts: ME "Router index"; C "Input FIFO size in flits"; D "Routing and arbitration delay"; F "Clock Frequency"; S "Standard Deviation"
      mask DialogControl DescGroupVar Prompt: XY Router
      mask DialogControl DescTextVar Prompt: 5 Port router with the XY routing algorithm.
  Router15 : Subsystem  mask{ME=15, C=1, D=1, F=1, S=1e-6}
      mask prompts: ME "Router index"; C "Input FIFO size in flits"; D "Routing and arbitration delay"; F "Clock Frequency"; S "Standard Deviation"
      mask DialogControl DescGroupVar Prompt: XY Router
      mask DialogControl DescTextVar Prompt: 5 Port router with the XY routing algorithm.
  Router16 : Subsystem  mask{ME=16, C=1, D=1, F=1, S=1e-6}
      mask prompts: ME "Router index"; C "Input FIFO size in flits"; D "Routing and arbitration delay"; F "Clock Frequency"; S "Standard Deviation"
      mask DialogControl DescGroupVar Prompt: XY Router
      mask DialogControl DescTextVar Prompt: 5 Port router with the XY routing algorithm.
  Router2 : Subsystem  mask{ME=2, C=1, D=1, F=1, S=1e-6}
      mask prompts: ME "Router index"; C "Input FIFO size in flits"; D "Routing and arbitration delay"; F "Clock Frequency"; S "Standard Deviation"
      mask DialogControl DescGroupVar Prompt: XY Router
      mask DialogControl DescTextVar Prompt: 5 Port router with the XY routing algorithm.
  Router3 : Subsystem  mask{ME=3, C=1, D=1, F=1, S=1e-6}
      mask prompts: ME "Router index"; C "Input FIFO size in flits"; D "Routing and arbitration delay"; F "Clock Frequency"; S "Standard Deviation"
      mask DialogControl DescGroupVar Prompt: XY Router
      mask DialogControl DescTextVar Prompt: 5 Port router with the XY routing algorithm.
  Router4 : Subsystem  mask{ME=4, C=1, D=1, F=1, S=1e-6}
      mask prompts: ME "Router index"; C "Input FIFO size in flits"; D "Routing and arbitration delay"; F "Clock Frequency"; S "Standard Deviation"
      mask DialogControl DescGroupVar Prompt: XY Router
      mask DialogControl DescTextVar Prompt: 5 Port router with the XY routing algorithm.
  Router5 : Subsystem  mask{ME=5, C=1, D=1, F=1, S=1e-6}
      mask prompts: ME "Router index"; C "Input FIFO size in flits"; D "Routing and arbitration delay"; F "Clock Frequency"; S "Standard Deviation"
      mask DialogControl DescGroupVar Prompt: XY Router
      mask DialogControl DescTextVar Prompt: 5 Port router with the XY routing algorithm.
  Router6 : Subsystem  mask{ME=6, C=1, D=1, F=1, S=1e-6}
      mask prompts: ME "Router index"; C "Input FIFO size in flits"; D "Routing and arbitration delay"; F "Clock Frequency"; S "Standard Deviation"
      mask DialogControl DescGroupVar Prompt: XY Router
      mask DialogControl DescTextVar Prompt: 5 Port router with the XY routing algorithm.
  Router7 : Subsystem  mask{ME=7, C=1, D=1, F=1, S=1e-6}
      mask prompts: ME "Router index"; C "Input FIFO size in flits"; D "Routing and arbitration delay"; F "Clock Frequency"; S "Standard Deviation"
      mask DialogControl DescGroupVar Prompt: XY Router
      mask DialogControl DescTextVar Prompt: 5 Port router with the XY routing algorithm.
  Router8 : Subsystem  mask{ME=8, C=1, D=1, F=1, S=1e-6}
      mask prompts: ME "Router index"; C "Input FIFO size in flits"; D "Routing and arbitration delay"; F "Clock Frequency"; S "Standard Deviation"
      mask DialogControl DescGroupVar Prompt: XY Router
      mask DialogControl DescTextVar Prompt: 5 Port router with the XY routing algorithm.
  Router9 : Subsystem  mask{ME=9, C=1, D=1, F=1, S=1e-6}
      mask prompts: ME "Router index"; C "Input FIFO size in flits"; D "Routing and arbitration delay"; F "Clock Frequency"; S "Standard Deviation"
      mask DialogControl DescGroupVar Prompt: XY Router
      mask DialogControl DescTextVar Prompt: 5 Port router with the XY routing algorithm.
  connections:
  Router1/RConn3 -- Router2/LConn2
  Router2/RConn2 -- Router1/LConn3
  Router2/RConn3 -- Router3/LConn2
  Router3/RConn2 -- Router2/LConn3
  Router3/RConn3 -- Router4/LConn2
  Router4/RConn2 -- Router3/LConn3
  Router5/RConn3 -- Router6/LConn2
  Router6/RConn2 -- Router5/LConn3
  Router6/RConn3 -- Router7/LConn2
  Router7/RConn2 -- Router6/LConn3
  Router7/RConn3 -- Router8/LConn2
  Router8/RConn2 -- Router7/LConn3
  Router9/RConn3 -- Router10/LConn2
  Router10/RConn2 -- Router9/LConn3
  Router10/RConn3 -- Router11/LConn2
  Router11/RConn2 -- Router10/LConn3
  Router11/RConn3 -- Router12/LConn2
  Router12/RConn2 -- Router11/LConn3
  Router13/RConn3 -- Router14/LConn2
  Router14/RConn2 -- Router13/LConn3
  Router14/RConn3 -- Router15/LConn2
  Router15/RConn2 -- Router14/LConn3
  Router15/RConn3 -- Router16/LConn2
  Router16/RConn2 -- Router15/LConn3
  Router1/RConn4 -- Router5/RConn1
  Router5/LConn1 -- Router1/LConn4
  Router5/RConn4 -- Router9/RConn1
  Router9/LConn1 -- Router5/LConn4
  Router9/RConn4 -- Router13/RConn1
  Router13/LConn1 -- Router9/LConn4
  Router2/RConn4 -- Router6/RConn1
  Router6/LConn1 -- Router2/LConn4
  Router6/RConn4 -- Router10/RConn1
  Router10/LConn1 -- Router6/LConn4
  Router10/RConn4 -- Router14/RConn1
  Router14/LConn1 -- Router10/LConn4
  Router3/RConn4 -- Router7/RConn1
  Router7/LConn1 -- Router3/LConn4
  Router7/RConn4 -- Router11/RConn1
  Router11/LConn1 -- Router7/LConn4
  Router11/RConn4 -- Router15/RConn1
  Router15/LConn1 -- Router11/LConn4
  Router4/RConn4 -- Router8/RConn1
  Router8/LConn1 -- Router4/LConn4
  Router8/RConn4 -- Router12/RConn1
  Router12/LConn1 -- Router8/LConn4
  Router12/RConn4 -- Router16/RConn1
  Router16/LConn1 -- Router12/LConn4
  PE1/LConn1 -- Router1/RConn5
  PE1/RConn1 -- Router1/LConn5
  PE2/LConn1 -- Router2/RConn5
  PE2/RConn1 -- Router2/LConn5
  PE3/LConn1 -- Router3/RConn5
  PE3/RConn1 -- Router3/LConn5
  PE4/LConn1 -- Router4/RConn5
  PE4/RConn1 -- Router4/LConn5
  PE5/LConn1 -- Router5/RConn5
  PE5/RConn1 -- Router5/LConn5
  PE6/LConn1 -- Router6/RConn5
  PE6/RConn1 -- Router6/LConn5
  PE7/LConn1 -- Router7/RConn5
  PE7/RConn1 -- Router7/LConn5
  PE8/LConn1 -- Router8/RConn5
  PE8/RConn1 -- Router8/LConn5
  PE9/LConn1 -- Router9/RConn5
  PE9/RConn1 -- Router9/LConn5
  PE10/LConn1 -- Router10/RConn5
  PE10/RConn1 -- Router10/LConn5
  PE11/LConn1 -- Router11/RConn5
  PE11/RConn1 -- Router11/LConn5
  PE12/LConn1 -- Router12/RConn5
  PE12/RConn1 -- Router12/LConn5
  PE13/LConn1 -- Router13/RConn5
  PE13/RConn1 -- Router13/LConn5
  PE14/LConn1 -- Router14/RConn5
  PE14/RConn1 -- Router14/LConn5
  PE15/LConn1 -- Router15/RConn5
  PE15/RConn1 -- Router15/LConn5
  PE16/LConn1 -- Router16/RConn5
  PE16/RConn1 -- Router16/LConn5

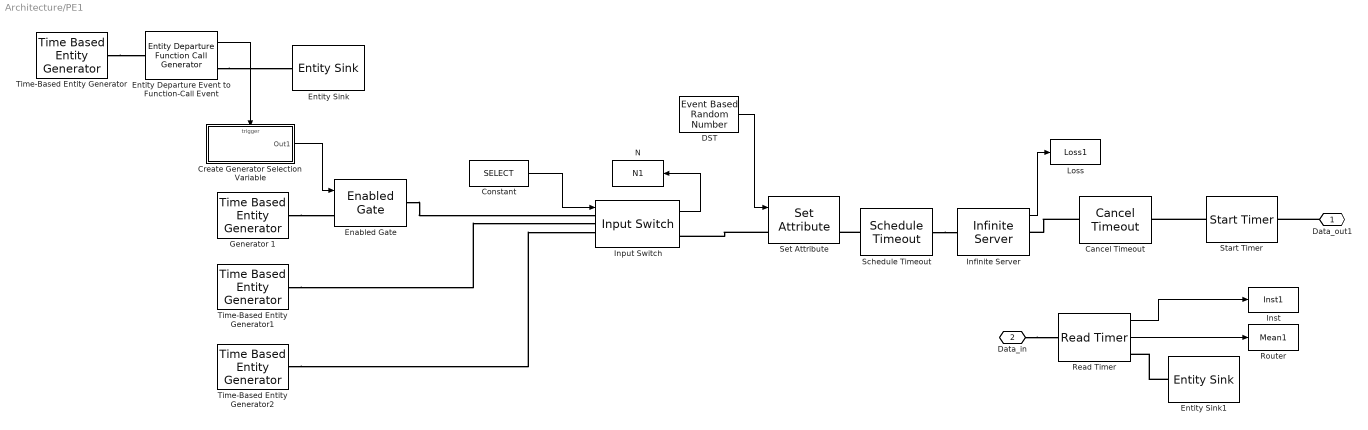
== system Architecture/PE1 ==
  Cancel Timeout : CancelTimeout
  Constant : Constant  Value=SELECT
  Create Generator Selection Variable : Subsystem  TreatAsAtomicUnit=on
  DST : EventBasedRandomNumber  Distribution=Arbitrary discrete  minUnid=1  maxUnid=16  numValueUnid=5  valueVecDisc=V  probVecDisc=P  Seed=SEED+5
  Enabled Gate : EnabledGate
  Entity Departure Event to Function-Call Event : EntityDepartureFunctionCallGenerator
  Entity Sink : EntitySink
  Entity Sink1 : EntitySink
  Generator 1 : TimeBasedEntityGenerator  Distribution=Exponential  Period=.1  InitialSeed=SEED+10  Maximum=.2  Mean=B  ResponseWhenUnblocked=Delayed restart  EntityType=Standard
  Infinite Server : InfiniteServer  ServiceTime=D  EnableTOPort=on  StatNumberTimedout=on
      settings: OutputPortMap=o5
  Input Switch : InputSwitch  NumberInputPorts=4  SwitchingCriterion=From signal port p  StatNumberDeparted=on
  Inst : ToWorkspace  VariableName=Inst1  SaveFormat=Timeseries  SampleTime=-1
  Loss : ToWorkspace  VariableName=Loss1  SaveFormat=Timeseries  SampleTime=-1
  N : ToWorkspace  VariableName=N1  SaveFormat=Timeseries  SampleTime=-1
  Read Timer : ReadTimer  TimerTag=Departure  StatTimeElapsed=on  StatAverageTimeElapsed=on
      settings: OutputPortMap=o2,o3
  Router : ToWorkspace  VariableName=Mean1  SaveFormat=Timeseries  SampleTime=-1
  Schedule Timeout : ScheduleTimeout  TimeoutInterval=D
  Set Attribute : SetAttribute  AttributeName=DST|SRC  AttributeFrom=Signal port|Dialog  AttributeValue=16|1  AttributeTreatAsVector=0|0  StatNumberDeparted=on  EvaluatedAttributeValue={ [];1}
  Start Timer : StartTimer  TimerTag=Departure
  Time-Based Entity Generator : TimeBasedEntityGenerator  Distribution=Exponential  Period=15  InitialSeed=SEED  Maximum=2  Mean=A  PriorityEntityGeneration=350  EntityType=Standard
  Time-Based Entity Generator1 : TimeBasedEntityGenerator  Period=REGULAR
  Time-Based Entity Generator2 : TimeBasedEntityGenerator  Distribution=Uniform  InitialSeed=SEED  Minimum=MINU  Maximum=MAXU
  Data_out1 : PMIOPort  Side=Right
  Data_in : PMIOPort  Port=2  Side=Left
  wires:
  DST/1 -> Set Attribute/1
  Infinite Server/1 -> Loss/1
  Input Switch/1 -> N/1
  Read Timer/2 -> Router/1
  Read Timer/1 -> Inst/1
  Constant/1 -> Input Switch/1
  Entity Departure Event to Function-Call Event/1 -> Create Generator Selection Variable/Trigger
  Create Generator Selection Variable/1(Out1) -> Enabled Gate/1
  connections:
  Enabled Gate/RConn1 -- Input Switch/LConn1
  Time-Based Entity Generator1/RConn1 -- Input Switch/LConn2
  Time-Based Entity Generator2/RConn1 -- Input Switch/LConn3
  Schedule Timeout/RConn1 -- Infinite Server/LConn1
  Data_in/RConn1 -- Read Timer/LConn1
  Entity Sink1/LConn1 -- Read Timer/RConn1
  Start Timer/LConn1 -- Cancel Timeout/RConn1
  Data_out1/RConn1 -- Start Timer/RConn1
  Set Attribute/LConn1 -- Input Switch/RConn1
  Cancel Timeout/LConn1 -- Infinite Server/RConn1
  Schedule Timeout/LConn1 -- Set Attribute/RConn1
  Generator 1/RConn1 -- Enabled Gate/LConn1
  Time-Based Entity Generator/RConn1 -- Entity Departure Event to Function-Call Event/LConn1
  Entity Departure Event to Function-Call Event/RConn1 -- Entity Sink/LConn1
